simulink library "osqp_library_base"  (Simulink 8.6)
settings: Solver=ode45  SolverMode=SingleTasking  StartTime=0.0  StopTime=10.0  RelTol=1e-3
values from neighbouring files (symbols this model uses):
  A = block.DialogPrm(4).Data    [osqp_sfun.m]
  l = max(l, osqp.constant('OSQP_INFTY'))    [osqp_sfun.m]
  P = block.DialogPrm(3).Data    [osqp_sfun.m]
  q = block.DialogPrm(5).Data    [osqp_sfun.m]
undefined symbols (not defined in the file or in its folder): osqp
settings Model: Creator=pgoulart  LastModifiedBy=imcinerney

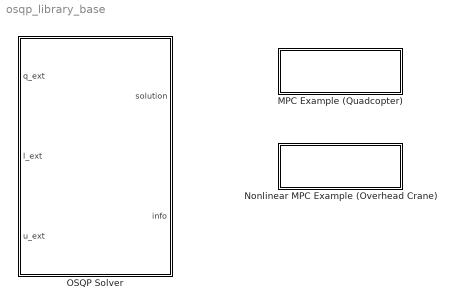
== system osqp_library_base ==
  MPC Example (Quadcopter) : Subsystem
      settings: OpenFcn=open_system('quadcopter_example','force');
      mask Display: disp('MPC Example\n(Quadcopter)')
  Nonlinear MPC Example (Overhead Crane) : Subsystem
      settings: OpenFcn=open_system('nonlinear_crane_example','force');
      mask Display: disp('Nonlinear MPC Example\n(Overhead Crane)')
  OSQP Solver : Subsystem  TreatAsAtomicUnit=on  mask(OSQP){P=P, A=A, q=q, l=l, u=u, opts={'verbose',true}, refactor_style=Never, warmstart_style=Always, has_external_q_input=on, has_external_bound_input=on, use_custom_osqp_dir=off, dirText=''}
      mask prompts: opts "OSQP Settings"; refactor_style "Refactorisation"; warmstart_style "Warm starting"; has_external_q_input "External linear cost (q)"; has_external_bound_input "External bounds (l,u)"; use_custom_osqp_dir "Export generated code to custom location"
      mask help: This block implements an OSQP solver object.
      mask init:
      | osqp_block_init(gcb)
      settings: RTWSystemCode=Nonreusable function
      mask TypeOptions refactor_style: Never | Always | Triggered
      mask TypeOptions warmstart_style: Never | Always | Triggered
      mask Callback use_custom_osqp_dir:
      | %p = Simulink.Mask.get( gcb );
      | %chkbox = p.Parameters( 11 )
      | %locBut = p.getDialogControl( 'location_button' );
      | %locBox = p.Parameters( 12 );
      | 
      | %enab = chkbox.Value;
      | %locBut.Visible = enab;
      | %locBox.Visible = enab;
      mask DialogControl use_custom_osqp_dir Tooltip: Export the code to a custom directory instead of the default
      mask DialogControl location_button Prompt: Change Location
      mask DialogControl location_button Callback:
      | p = Simulink.Mask.get( gcb );
      | dirTxt = p.Parameters( 12 );
      | 
      | selpath = uigetdir( pwd, 'Select directory to export OSQP code to' );
      | dirTxt.Value = ['''', selpath, ''''];

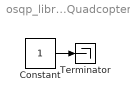
== system osqp_library_base/MPC Example (Quadcopter) ==
  Constant : Constant
  Terminator : Terminator
  wires:
  Constant/1 -> Terminator/1

== system osqp_library_base/Nonlinear MPC Example (Overhead Crane) ==

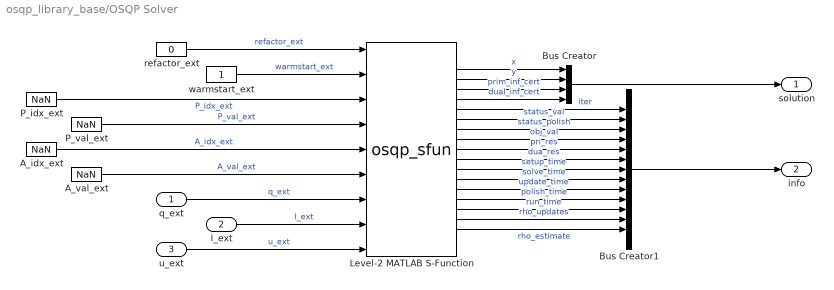
== system osqp_library_base/OSQP Solver ==
  q_ext : Inport
  l_ext : Inport  Port=2
  u_ext : Inport  Port=3
  A_idx_ext : Constant  Value=NaN
  A_val_ext : Constant  Value=NaN
  Bus Creator : BusCreator  Inputs=4
  Bus Creator1 : BusCreator  Inputs=13
  Level-2 MATLAB S-Function : M-S-Function  FunctionName=osqp_sfun  Parameters=size(A,1),size(A,2),P,A,q,l,u,osqp,opts
  P_idx_ext : Constant  Value=NaN
  P_val_ext : Constant  Value=NaN
  refactor_ext : Constant  Value=0
  warmstart_ext : Constant
  solution : Outport
  info : Outport  Port=2
  wires:
  warmstart_ext/1 -> Level-2 MATLAB S-Function/2  "warmstart_ext"
  l_ext/1 -> Level-2 MATLAB S-Function/8  "l_ext"
  A_idx_ext/1 -> Level-2 MATLAB S-Function/5  "A_idx_ext"
  P_idx_ext/1 -> Level-2 MATLAB S-Function/3  "P_idx_ext"
  Level-2 MATLAB S-Function/8 -> Bus Creator1/4  "obj_val"
  Level-2 MATLAB S-Function/15 -> Bus Creator1/11  "run_time"
  u_ext/1 -> Level-2 MATLAB S-Function/9  "u_ext"
  Level-2 MATLAB S-Function/9 -> Bus Creator1/5  "pri_res"
  Level-2 MATLAB S-Function/17 -> Bus Creator1/13  "rho_estimate"
  P_val_ext/1 -> Level-2 MATLAB S-Function/4  "P_val_ext"
  A_val_ext/1 -> Level-2 MATLAB S-Function/6  "A_val_ext"
  refactor_ext/1 -> Level-2 MATLAB S-Function/1  "refactor_ext"
  q_ext/1 -> Level-2 MATLAB S-Function/7  "q_ext"
  Level-2 MATLAB S-Function/12 -> Bus Creator1/8  "solve_time"
  Level-2 MATLAB S-Function/1 -> Bus Creator/1  "x"
  Level-2 MATLAB S-Function/4 -> Bus Creator/4  "dual_inf_cert"
  Level-2 MATLAB S-Function/2 -> Bus Creator/2  "y"
  Level-2 MATLAB S-Function/3 -> Bus Creator/3  "prim_inf_cert"
  Level-2 MATLAB S-Function/6 -> Bus Creator1/2  "status_val"
  Level-2 MATLAB S-Function/11 -> Bus Creator1/7  "setup_time"
  Level-2 MATLAB S-Function/14 -> Bus Creator1/10  "polish_time"
  Level-2 MATLAB S-Function/5 -> Bus Creator1/1  "iter"
  Level-2 MATLAB S-Function/7 -> Bus Creator1/3  "status_polish"
  Level-2 MATLAB S-Function/16 -> Bus Creator1/12  "rho_updates"
  Level-2 MATLAB S-Function/13 -> Bus Creator1/9  "update_time"
  Level-2 MATLAB S-Function/10 -> Bus Creator1/6  "dua_res"
  Bus Creator/1 -> solution/1
  Bus Creator1/1 -> info/1
